simulink model "Labi_project1"  (R2017a)
settings: Solver=VariableStepAuto  StartTime=0.0  StopTime=10.0  RelTol=1e-3
settings Model: Creator=DoktorHax  LastModifiedBy=DoktorHax

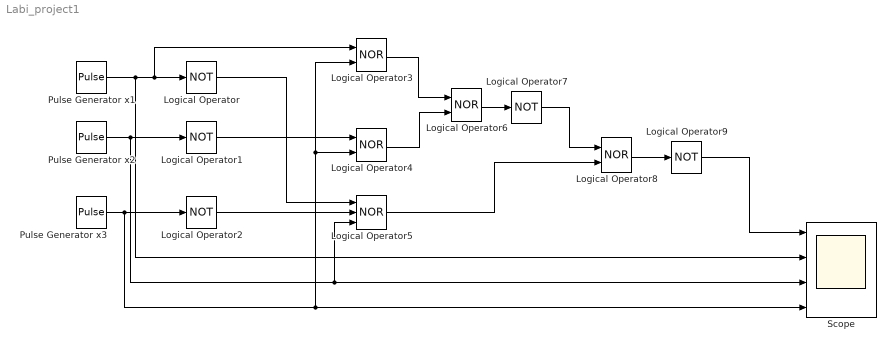
== system Labi_project1 ==
  Logical Operator{,1..2,7,9} (5 alike) : Logic  Operator=NOT  AllPortsSameDT=off  OutDataTypeStr=boolean
  Logical Operator{3..4,6,8} (4 alike) : Logic  Operator=NOR  AllPortsSameDT=off  OutDataTypeStr=boolean
  Logical Operator5 : Logic  Operator=NOR  Inputs=3  AllPortsSameDT=off  OutDataTypeStr=boolean
  Pulse Generator x1 : DiscretePulseGenerator  PulseType=Time based  PulseWidth=50
  Pulse Generator x2 : DiscretePulseGenerator  PulseType=Time based  Period=4  PulseWidth=50
  Pulse Generator x3 : DiscretePulseGenerator  PulseType=Time based  Period=8  PulseWidth=50
  Scope : Scope  NumInputPorts=4
  wires:
  Pulse Generator x1/1 -> Logical Operator3/1, Logical Operator/1, Scope/2
  Pulse Generator x2/1 -> Logical Operator5/3, Scope/3, Logical Operator1/1
  Logical Operator/1 -> Logical Operator5/1
  Logical Operator2/1 -> Logical Operator5/2
  Logical Operator1/1 -> Logical Operator4/1
  Logical Operator3/1 -> Logical Operator6/1
  Logical Operator4/1 -> Logical Operator6/2
  Logical Operator6/1 -> Logical Operator7/1
  Logical Operator7/1 -> Logical Operator8/1
  Logical Operator8/1 -> Logical Operator9/1
  Logical Operator9/1 -> Scope/1
  Logical Operator5/1 -> Logical Operator8/2
  Pulse Generator x3/1 -> Logical Operator4/2, Logical Operator3/2, Scope/4, Logical Operator2/1
